simulink model "b_node2"  (R2012b)
settings: Solver=FixedStepDiscrete  SolverMode=SingleTasking  StartTime=0.0  StopTime=inf  RelTol=1e-3
model workspace (MAT data in the model file):
  lambda = Simulink.Parameter
  lambda.DataType = 'auto'
libraries: simulink x2
settings Model: Creator=andreas  LastModifiedBy=andreas
settings DataIOCC: SaveOutput=off  SignalLogging=off  SaveTime=off
settings OptimizationCC: InlineParams=on
settings DebuggingCC: AlgebraicLoopMsg=error  SingleTaskRateTransMsg=error
settings ModelReferenceCC: UpdateModelReferenceTargets=IfOutOfDate

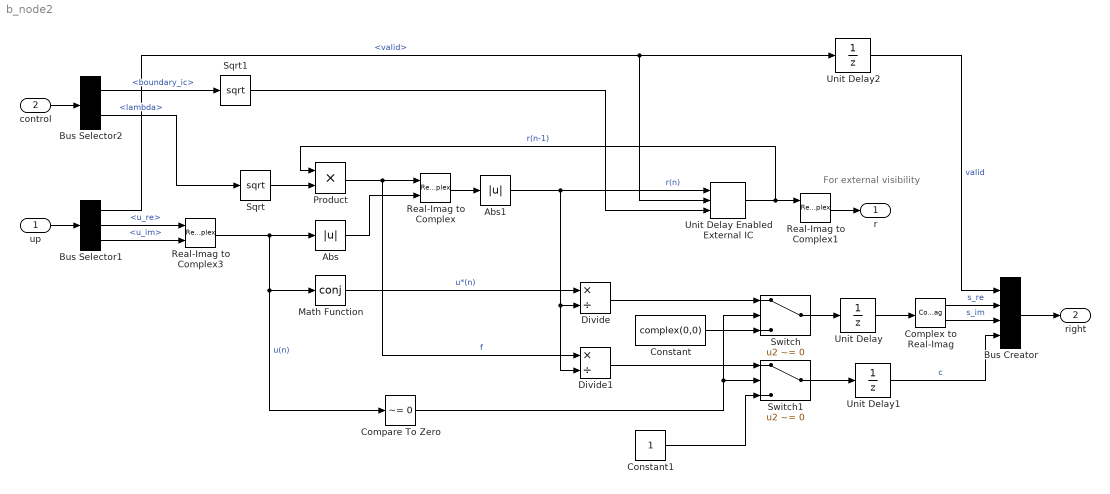
== system b_node2 ==
  note: For external
      | visibility
  up : Inport  OutDataTypeStr=Bus: vbus
  control : Inport  Port=2  OutDataTypeStr=Bus: cbus
  Abs : Abs
  Abs1 : Abs
  Bus Creator : BusCreator
  Bus Selector1 : BusSelector  OutputSignals=valid,u_re,u_im
  Bus Selector2 : BusSelector  OutputSignals=boundary_ic,lambda
  Compare To Zero : simulink/Logic and Bit Operations/Compare To Zero  relop=~=  OutDataTypeStr=boolean
  Complex to Real-Imag : ComplexToRealImag
  Constant : Constant  Value=complex(0,0)  OutDataTypeStr=Inherit: Inherit via back propagation
  Constant1 : Constant
  Divide : Product  Inputs=*/
  Divide1 : Product  Inputs=*/
  Math Function : Math  Operator=conj  SaturateOnIntegerOverflow=on
  Product : Product  RndMeth=Zero
  Real-Imag to Complex : RealImagToComplex
  Real-Imag to Complex1 : RealImagToComplex
  Real-Imag to Complex3 : RealImagToComplex
  Sqrt : Sqrt  SaturateOnIntegerOverflow=on
  Sqrt1 : Sqrt  SaturateOnIntegerOverflow=on
  Switch : Switch  Criteria=u2 ~= 0
  Switch1 : Switch  Criteria=u2 ~= 0
  Unit Delay : UnitDelay  SampleTime=-1
  Unit Delay Enabled External IC : simulink/Additional Math & Discrete/Additional Discrete/Unit Delay Enabled External IC  tsamp=-1
  Unit Delay1 : UnitDelay  SampleTime=-1
  Unit Delay2 : UnitDelay  SampleTime=-1
  r : Outport
      settings: SignalType=complex
  right : Outport  Port=2  OutDataTypeStr=Bus: hbus
      settings: SignalType=complex
  wires:
  Sqrt/1 -> Product/2
  Real-Imag to Complex3/1 -> Compare To Zero/1, Math Function/1, Abs/1  "u(n)"
  Abs1/1 -> Divide/2, Divide1/2, Unit Delay Enabled External IC/1  "r(n)"
  Unit Delay Enabled External IC/1 -> Product/1, Real-Imag to Complex1/1  "r(n-1)"
  Abs/1 -> Real-Imag to Complex/2
  Product/1 -> Real-Imag to Complex/1, Divide1/1  "f"
  Real-Imag to Complex/1 -> Abs1/1
  Unit Delay1/1 -> Bus Creator/4  "c"
  Math Function/1 -> Divide/1  "u*(n)"
  Real-Imag to Complex1/1 -> r/1
  Sqrt1/1 -> Unit Delay Enabled External IC/3
  Divide/1 -> Switch/1
  Switch/1 -> Unit Delay/1
  Divide1/1 -> Switch1/1
  Switch1/1 -> Unit Delay1/1
  Compare To Zero/1 -> Switch/2, Switch1/2
  Constant/1 -> Switch/3
  Constant1/1 -> Switch1/3
  Bus Selector1/1 -> Unit Delay2/1, Unit Delay Enabled External IC/2  "<valid>"
  Bus Selector1/2 -> Real-Imag to Complex3/1  "<u_re>"
  Bus Selector1/3 -> Real-Imag to Complex3/2  "<u_im>"
  up/1 -> Bus Selector1/1
  Unit Delay/1 -> Complex to Real-Imag/1
  Complex to Real-Imag/1 -> Bus Creator/2  "s_re"
  Complex to Real-Imag/2 -> Bus Creator/3  "s_im"
  Bus Creator/1 -> right/1
  Unit Delay2/1 -> Bus Creator/1  "valid"
  control/1 -> Bus Selector2/1
  Bus Selector2/1 -> Sqrt1/1  "<boundary_ic>"
  Bus Selector2/2 -> Sqrt/1  "<lambda>"
